simulink library "DYN_MAG"  (Simulink 10.1)
settings: Solver=VariableStepAuto  StartTime=0.0  StopTime=10.0  RelTol=1e-3
undefined symbols (not defined in the file): IAU
libraries: LIB_ROT x5, vrlib x1, aerolibtransform2 x1, aerolibgravity2 x1
settings Model: Creator=WilTravis  LastModifiedBy=m_mam

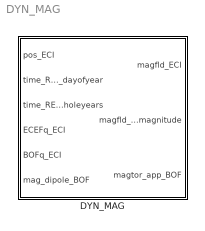
== system DYN_MAG ==
  DYN_MAG : Subsystem

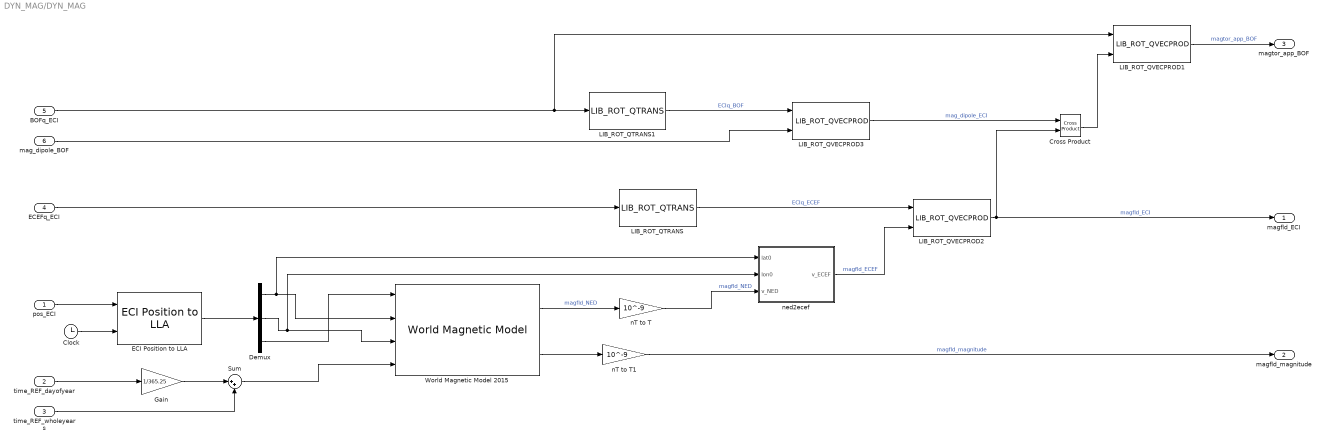
== system DYN_MAG/DYN_MAG ==
  pos_ECI : Inport
  time_REF_dayofyear : Inport  Port=2
  time_REF_wholeyears : Inport  Port=3
  ECEFq_ECI : Inport  Port=4
  BOFq_ECI : Inport  Port=5
  mag_dipole_BOF : Inport  Port=6
  Clock : Clock
  Cross Product : vrlib/Utilities/Cross Product
  Demux : Demux  Outputs=3
  ECI Position to LLA : aerolibtransform2/ECI Position to LLA  red=IAU-2000/2006  year=2018  month=January  day=1  hour=0  min=0  sec=0  deltaT=Sec  errorflag=Error  extraparamflag=off  eunits=Metric (MKS)  earthmodel=WGS84  flat=1/298.257223563  eqradius=6378137
      settings: AttributesFormatString=%<red>  SourceProductBaseCode=AE
  Gain : Gain  Gain=1/365.25
  LIB_ROT_QTRANS : LIB_ROT/LIB_ROT_QTRANS
  LIB_ROT_QTRANS1 : LIB_ROT/LIB_ROT_QTRANS
  LIB_ROT_QVECPROD1 : LIB_ROT/LIB_ROT_QVECPROD
  LIB_ROT_QVECPROD2 : LIB_ROT/LIB_ROT_QVECPROD
  LIB_ROT_QVECPROD3 : LIB_ROT/LIB_ROT_QVECPROD
  Sum : Sum  Inputs=|++
  World Magnetic Model 2015 : aerolibgravity2/World Magnetic Model  model=WMM2015 V2 (2015-2020)  customFile='WMM2020.COF'  units=Metric (MKS)  time_in=on  month=January  day=1  year=2015  action=Warning  h_out=off  dec_out=off  inc_out=off  ti_out=on
      settings: SourceProductBaseCode=AE
  nT to T : Gain  Gain=10^-9
  nT to T1 : Gain  Gain=10^-9
  ned2ecef : MATLAB Function  TreatAsAtomicUnit=on
  magfld_ECI : Outport  VectorParamsAs1DForOutWhenUnconnected=off
  magfld_magnitude : Outport  Port=2  VectorParamsAs1DForOutWhenUnconnected=off
  magtor_app_BOF : Outport  Port=3  VectorParamsAs1DForOutWhenUnconnected=off
  wires:
  pos_ECI/1 -> ECI Position to LLA/1
  ECEFq_ECI/1 -> LIB_ROT_QTRANS/1
  LIB_ROT_QTRANS/1 -> LIB_ROT_QVECPROD2/1  "ECIq_ECEF"
  LIB_ROT_QVECPROD2/1 -> Cross Product/2, magfld_ECI/1  "magfld_ECI"
  BOFq_ECI/1 -> LIB_ROT_QVECPROD1/1, LIB_ROT_QTRANS1/1
  World Magnetic Model 2015/1 -> nT to T/1  "magfld_NED"
  ECI Position to LLA/1 -> Demux/1
  World Magnetic Model 2015/2 -> nT to T1/1
  Cross Product/1 -> LIB_ROT_QVECPROD1/2
  nT to T1/1 -> magfld_magnitude/1  "magfld_magnitude"
  time_REF_dayofyear/1 -> Gain/1
  LIB_ROT_QTRANS1/1 -> LIB_ROT_QVECPROD3/1  "ECIq_BOF"
  mag_dipole_BOF/1 -> LIB_ROT_QVECPROD3/2
  LIB_ROT_QVECPROD3/1 -> Cross Product/1  "mag_dipole_ECI"
  Gain/1 -> Sum/1
  time_REF_wholeyears/1 -> Sum/2
  Sum/1 -> World Magnetic Model 2015/4
  Clock/1 -> ECI Position to LLA/2
  LIB_ROT_QVECPROD1/1 -> magtor_app_BOF/1  "magtor_app_BOF"
  ned2ecef/1(v_ECEF) -> LIB_ROT_QVECPROD2/2  "magfld_ECEF"
  nT to T/1 -> ned2ecef/3(v_NED)  "magfld_NED"
  Demux/3 -> World Magnetic Model 2015/1
  Demux/1 -> ned2ecef/1(lat0), World Magnetic Model 2015/2
  Demux/2 -> ned2ecef/2(lon0), World Magnetic Model 2015/3

== matlab function DYN_MAG/ned2ecef ==
  data: lat0 input double; lon0 input double; v_NED input double; v_ECEF output double
function v_ECEF  = ned2ecef(lat0, lon0, v_NED)
%NED2ECEFV Rotate vector from local NED to ECEF
%
%   [U, V, W] = NED2ECEFV(uNorth, vEast, wDown, LAT0, LON0) rotates a
%   Cartesian 3-vector with components uNorth, vEast, wDown from a local
%   north-east-down (NED) system with origin at latitude LAT0 and longitude
%   LON0 to a geocentric Earth-Centered, Earth-Fixed (ECEF) system. The
%   origin latitude and longitude are assumed to be in units of degrees.
%
%   [...] = NED2ECEFV(..., angleUnit) uses angleUnit, which matches either
%   'degrees' or 'radians', to specify the units of the local origin
%   latitude and longitude.
%
%   To transform coordinate locations instead of vectors, use the ned2ecef
%   function.
%
%   Class support for vector components and angles:
%      float: double, single
%
%   See also ENU2ECEFV, ECEF2ENUV, ECEF2NEDV

% Copyright 2012-2019 The MathWorks, Inc.

uNorth = v_NED(1);
vEast = v_NED(2);
wDown = v_NED(3);

sinfun = @sind;
cosfun = @cosd;

uEast = vEast;
vNorth = uNorth;
wUp = -wDown;

cosPhi = cosfun(lat0);
sinPhi = sinfun(lat0);
cosLambda = cosfun(lon0);
sinLambda = sinfun(lon0);

t = cosPhi .* wUp - sinPhi .* vNorth;
w = sinPhi .* wUp + cosPhi .* vNorth;

u = cosLambda .* t - sinLambda .* uEast;
v = sinLambda .* t + cosLambda .* uEast;

v_ECEF = [u; v; w];
